simulink model "positionControlLoopCircle"  (Simulink 7.5)
settings: Solver=FixedStepDiscrete  StartTime=0.0  StopTime=Inf  FixedStep=Ts  RelTol=1e-3
PostLoadFcn:
  | , if any(exist('dsrtsu_mdlpostloadfcn', 'file') == [2, 3, 6]), try dsrtsu_mdlpostloadfcn('Execute', bdroot); catch fprintf('Error in PostLoadFcn (dsrtsu_mdlpostloadfcn) for model "%s":\n %s\n', bdroot, lasterr); end, end,
values from neighbouring files (symbols this model uses):
  Bx = 0.002015920056936    (= 0.00201592005694)    [main.m]
  By = 8.925446348616319e-004    (= 0.000892544634862)    [main.m]
  center = [xc;yc]    [main.m]    (also in main2.m)
  circX = center(1)+rad*cos(theta)    [genCircle.m]    (also in main.m = circXt(1:floor(length(circXt))); main2.m = circX(1:floor(length(circX)/factor)))
  circY = center(2)+rad*sin(theta)    [genCircle.m]    (also in main.m = circYt(1:floor(length(circYt))); main2.m = circY(1:floor(length(circY)/factor)))
  Jx = 9.170930148991473e-004    (= 0.000917093014899)    [main.m]
  Jy = 5.701918282653577e-004    (= 0.000570191828265)    [main.m]
  Ts = 0.01    [main.m]    (also in main2.m = 0.001)
  zeta = 0.8    [main.m]
undefined symbols (not defined in the file or in its folder): DiscIntNeverNeededParam
libraries: rtilib1103 x12, simulink x2
settings Model: DSRTSU_INTERNAL_RTI_VER=360  DSRTSU_INTERNAL_RTI_TYPE=rti1103  Creator=daq  LastModifiedBy=daq  BufferReuse=off
settings OptimizationCC: BlockReduction=off  OptimizeBlockIOStorage=off  BufferReuse=off  ExpressionFolding=off  LocalBlockOutputs=off
settings HardwareCC: ProdIntDivRoundTo=Zero  ProdEndianess=BigEndian  ProdHWDeviceType=Generic->Custom  TargetIntDivRoundTo=Zero  TargetEndianess=BigEndian  TargetHWDeviceType=Generic->Custom
settings RTWCC: SystemTargetFile=rti1103.tlc  MakeCommand=make_rti  TemplateMakefile=rti1103.tmf  Description=dSPACE DS1103 Hardware Platform  ProcessScript=rti1103_make_rtw_hook
settings STFCustomTargetCC: ParMdlRefBuildCompliant=on  GeneratePreprocessorConditionals=Disable all  SystemTargetFile=rti1103.tlc
settings GRTTargetCC: CompOptLevelCompliant=off  MatFileLogging=off  ExtModeMexFile=noextcomm
settings CustomProperty: DataType=RTWOptions_EnumType_C__dSPACE_matlab_rti1103_tlc_rti1103_1InitialSimState  Value=RUN
settings EnumStrPairs: String=RUN

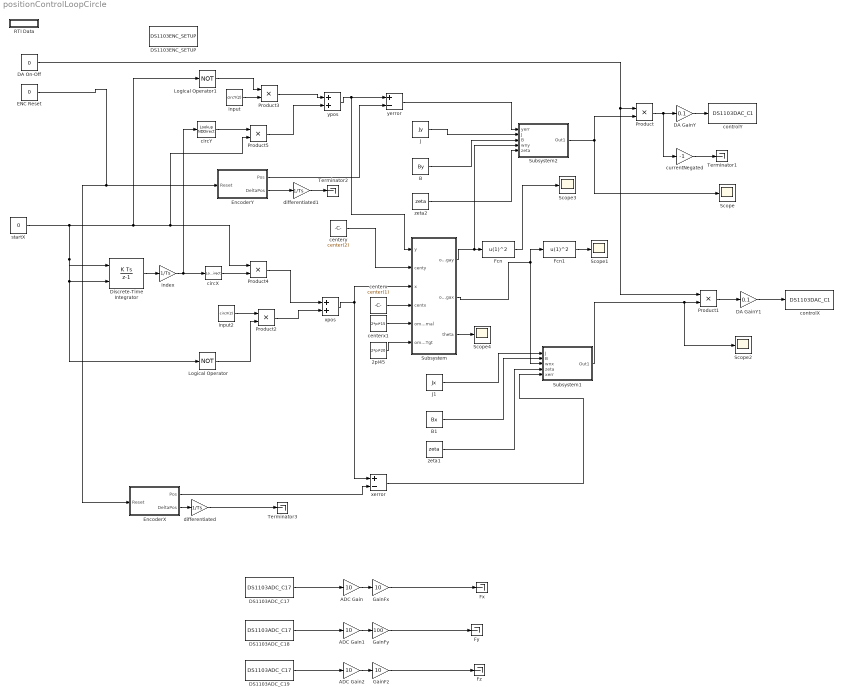
== system positionControlLoopCircle ==
  " EncoderX" : Subsystem
  " EncoderY" : Subsystem
  2pi45 : Constant  Value=2*pi*20  OutDataType=fixdt(1, 16)  OutScaling=2^0
  ADC Gain : Gain  Gain=10  ParameterDataType=fixdt(1, 16)  ParameterScaling=2^0  OutDataType=fixdt(1, 16)  OutScaling=2^0
  ADC Gain1 : Gain  Gain=10  ParameterDataType=fixdt(1, 16)  ParameterScaling=2^0  OutDataType=fixdt(1, 16)  OutScaling=2^0
  ADC Gain2 : Gain  Gain=10  ParameterDataType=fixdt(1, 16)  ParameterScaling=2^0  OutDataType=fixdt(1, 16)  OutScaling=2^0
  B : Constant  Value=By  OutDataType=fixdt(1, 16)  OutScaling=2^0
  B1 : Constant  Value=Bx  OutDataType=fixdt(1, 16)  OutScaling=2^0
  DA GainY : Gain  Gain=0.1  ParameterDataType=fixdt(1, 16)  ParameterScaling=2^0  OutDataType=fixdt(1, 16)  OutScaling=2^0
  DA GainY1 : Gain  Gain=0.1  ParameterDataType=fixdt(1, 16)  ParameterScaling=2^0  OutDataType=fixdt(1, 16)  OutScaling=2^0
  DA On-Off : Constant  Value=0  OutDataType=fixdt(1, 16)  OutScaling=2^0
  DS1103ADC_C17 : rtilib1103/DS1103 MASTER PPC/DS1103ADC_C17  SystemSampleTime=-1  ChannelNo=17  TimerAPreTrigger=0  Reserved2=[]  Reserved3=[]  Reserved4=[]  DialogFcn=gui1103adc  UnitName={ 'DS1103ADC_C' }  UnitValues={ 17 }  DSProperties=struct('RTI',struct('Version',uint32(1),'BlockType',struct('isSLSource',uint8(1),'isSLSink',uint8(0),'isHWSource',uint8(1),'isHWSink',uint8(0),'isSetup',uint8(0),'isInline',uint8(1),'isNonInline',uint8(0),'isInterrupt',uint8(0),'isChannelwise',uint8(1)),'IOBoardType','DS1103MASTER','UnitType','ADC','Identifier','ADC','DialogType','ML','BlockSet','NONE','SlaveProcessor','NONE'))
  DS1103ADC_C18 : rtilib1103/DS1103 MASTER PPC/DS1103ADC_C17  SystemSampleTime=-1  ChannelNo=18  TimerAPreTrigger=0  Reserved2=[]  Reserved3=[]  Reserved4=[]  DialogFcn=gui1103adc  UnitName={ 'DS1103ADC_C' }  UnitValues={ 18 }  DSProperties=struct('RTI',struct('Version',uint32(1),'BlockType',struct('isSLSource',uint8(1),'isSLSink',uint8(0),'isHWSource',uint8(1),'isHWSink',uint8(0),'isSetup',uint8(0),'isInline',uint8(1),'isNonInline',uint8(0),'isInterrupt',uint8(0),'isChannelwise',uint8(1)),'IOBoardType','DS1103MASTER','UnitType','ADC','Identifier','ADC','DialogType','ML','BlockSet','NONE','SlaveProcessor','NONE'))
  DS1103ADC_C19 : rtilib1103/DS1103 MASTER PPC/DS1103ADC_C17  SystemSampleTime=-1  ChannelNo=19  TimerAPreTrigger=0  Reserved2=[]  Reserved3=[]  Reserved4=[]  DialogFcn=gui1103adc  UnitName={ 'DS1103ADC_C' }  UnitValues={ 19 }  DSProperties=struct('RTI',struct('Version',uint32(1),'BlockType',struct('isSLSource',uint8(1),'isSLSink',uint8(0),'isHWSource',uint8(1),'isHWSink',uint8(0),'isSetup',uint8(0),'isInline',uint8(1),'isNonInline',uint8(0),'isInterrupt',uint8(0),'isChannelwise',uint8(1)),'IOBoardType','DS1103MASTER','UnitType','ADC','Identifier','ADC','DialogType','ML','BlockSet','NONE','SlaveProcessor','NONE'))
  DS1103ENC_SETUP : rtilib1103/DS1103 MASTER PPC/DS1103ENC_SETUP  SystemSampleTime=-1  EncRange=0  Reserved1=[]  Reserved2=[]  Reserved3=[]  Reserved4=[]  DialogFcn=gui1103enc_setup  UnitName={ 'DS1103ENC_SETUP' }  UnitValues={ [] }  DSProperties=struct('RTI',struct('Version',uint32(1),'BlockType',struct('isSLSource',uint8(0),'isSLSink',uint8(0),'isHWSource',uint8(0),'isHWSink',uint8(0),'isSetup',uint8(0),'isInline',uint8(1),'isNonInline',uint8(0),'isInterrupt',uint8(0),'isChannelwise',uint8(0)),'IOBoardType','DS1103MASTER','UnitType','ENC','Identifier','ENCMASTER','DialogType','ML','BlockSet','NONE','SlaveProcessor','NONE'))
      settings: SignalType=[0 0 0 0 0 0 0]
  Discrete-Time Integrator : DiscreteIntegrator  ExternalReset=rising  SampleTime=Ts  OutDataType=fixdt(1, 16)  OutScaling=2^0  ICPrevOutput=DiscIntNeverNeededParam  ICPrevScaledInput=DiscIntNeverNeededParam
  ENC Reset : Constant  Value=0  OutDataType=fixdt(1, 16)  OutScaling=2^0
  Fcn : Fcn  Expr=u(1)^2
  Fcn1 : Fcn  Expr=u(1)^2
  Fx : Terminator
  Fy : Terminator
  Fz : Terminator
  GainFx : Gain  Gain=10  ParameterDataType=fixdt(1, 16)  ParameterScaling=2^0  OutDataType=fixdt(1, 16)  OutScaling=2^0
  GainFy : Gain  Gain=100  ParameterDataType=fixdt(1, 16)  ParameterScaling=2^0  OutDataType=fixdt(1, 16)  OutScaling=2^0
  GainFz : Gain  Gain=10  ParameterDataType=fixdt(1, 16)  ParameterScaling=2^0  OutDataType=fixdt(1, 16)  OutScaling=2^0
  J : Constant  Value=Jy  OutDataType=fixdt(1, 16)  OutScaling=2^0
  J1 : Constant  Value=Jx  OutDataType=fixdt(1, 16)  OutScaling=2^0
  Logical Operator : Logic  Operator=NOT  AllPortsSameDT=off  OutDataTypeMode=boolean  LogicDataType=fixdt(0, 8)  OutDataTypeStr=boolean
  Logical Operator1 : Logic  Operator=NOT  AllPortsSameDT=off  OutDataTypeMode=boolean  LogicDataType=fixdt(0, 8)  OutDataTypeStr=boolean
  Product{,1..5} (6 alike) : Product  OutDataType=fixdt(1, 16)  OutScaling=2^0  RndMeth=Zero
  RTI Data : Subsystem  Tag=struct('RTIDataServer',struct('RTIDataServerVs','2','RTIModelDescription','struct(''main'',''positionControlLoopCircle'',''sub'','''',''isMp'',0)'))  LoadFcn="if exist('rtidc'), try,  rtidc('DataHostBlockClbLoad', gcbh); catch, disp(['Warning: ''LoadFcn'' for RTI Data block failed: ' lasterr]); end, end,"
      settings: CopyFcn="if exist('rtidc'), try,  rtidc('DataHostBlockClbCopy', gcbh); catch, disp(['Warning: ''CopyFcn'' for RTI Data block failed: ' lasterr]); end, end,"  DeleteFcn="if exist('rtidc'), try,  rtidc('DataHostBlockClbDelete', gcbh); catch, disp(['Warning: ''DeleteFcn'' for RTI Data block failed: ' lasterr]); end, end,"  ModelCloseFcn="if exist('rtidc'), try,  rtidc('DataHostBlockClbModelClose', gcbh); catch, disp(['Warning: ''ModelCloseFcn'' for RTI Data block failed: ' lasterr]); end, end,"  PreSaveFcn="if exist('rtidc'), try,  rtidc('DataHostBlockClbPreSave', gcbh); catch, disp(['Warning: ''PreSaveFcn'' for RTI Data block failed: ' lasterr]); end, end,"  PostSaveFcn="if exist('rtidc'), try,  rtidc('DataHostBlockClbPostSave', gcbh); catch, disp(['Warning: ''PostSaveFcn'' for RTI Data block failed: ' lasterr]); end, end,"  NameChangeFcn="if exist('rtidc'), try,  rtidc('DataHostBlockClbNameChange', gcbh); catch, disp(['Warning: ''NameChangeFcn'' for RTI Data block failed: ' lasterr]); end, end,"
      mask Type: RTI_DATA_HOST
      mask Description:
      | RTI Data Block.
      | This block is used by RTI to store internal model-dependent data.
      | Please keep this block on the root level of the model. Deleting this block will result in data loss.
      | 
      | NEVER DELETE OR COPY THIS BLOCK!
      mask Help:
      | RTI Data Block.
      | This block is used by RTI to store internal model-dependent data.
      | Please keep this block on the root level of the model. Deleting this block will result in data loss.
      | 
      | NEVER DELETE OR COPY THIS BLOCK!
      mask Display:
      | text(0.5, 0.5, 'RTI Data', 'HorizontalAlignment', 'center');
      | plot([1 0]);
  Scope{,1..4} (5 alike) : Scope
      Scope2 settings: SaveName=ScopeData2
      Scope3 settings: SaveName=ScopeData3
      Scope4 settings: SaveName=ScopeData4
  Subsystem : Subsystem
  Subsystem1 : Subsystem
  Subsystem2 : Subsystem
  Terminator1 : Terminator
  Terminator2 : Terminator
  Terminator3 : Terminator
  centerx : Constant  Value=center(1)  OutDataType=fixdt(1, 16)  OutScaling=2^0
  centerx1 : Constant  Value=2*pi*15  OutDataType=fixdt(1, 16)  OutScaling=2^0
  centery : Constant  Value=center(2)  OutDataType=fixdt(1, 16)  OutScaling=2^0
  circX : LookupNDDirect  NumberOfTableDimensions=1  Table=circX
  circY : LookupNDDirect  NumberOfTableDimensions=1  Table=circY
  controlX : rtilib1103/DS1103 MASTER PPC/DS1103DAC_C1  SystemSampleTime=-1  ChannelNo=1  InitValue=0  TermMode=0  TermValue=0  Reserved1=[]  Reserved2=[]  Reserved3=[]  Reserved4=[]  DialogFcn=gui1103dac  UnitName={ 'DS1103DAC_C' }  UnitValues={ 1 }  DSProperties=struct('RTI',struct('Version',uint32(1),'BlockType',struct('isSLSource',uint8(0),'isSLSink',uint8(1),'isHWSource',uint8(0),'isHWSink',uint8(1),'isSetup',uint8(0),'isInline',uint8(1),'isNonInline',uint8(0),'isInterrupt',uint8(0),'isChannelwise',uint8(1)),'IOBoardType','DS1103MASTER','UnitType','DAC','Identifier','DAC','DialogType','ML','BlockSet','NONE','SlaveProcessor','NONE'))
  controlY : rtilib1103/DS1103 MASTER PPC/DS1103DAC_C1  SystemSampleTime=-1  ChannelNo=2  InitValue=0  TermMode=1  TermValue=0  Reserved1=[]  Reserved2=[]  Reserved3=[]  Reserved4=[]  DialogFcn=gui1103dac  UnitName={ 'DS1103DAC_C' }  UnitValues={ 2 }  DSProperties=struct('RTI',struct('Version',uint32(1),'BlockType',struct('isSLSource',uint8(0),'isSLSink',uint8(1),'isHWSource',uint8(0),'isHWSink',uint8(1),'isSetup',uint8(0),'isInline',uint8(1),'isNonInline',uint8(0),'isInterrupt',uint8(0),'isChannelwise',uint8(1)),'IOBoardType','DS1103MASTER','UnitType','DAC','Identifier','DAC','DialogType','ML','BlockSet','NONE','SlaveProcessor','NONE'))
  currentNegated : Gain  Gain=-1  ParameterDataType=fixdt(1, 16)  ParameterScaling=2^0  OutDataType=fixdt(1, 16)  OutScaling=2^0
  differentiated : Gain  Gain=1/Ts  ParameterDataType=fixdt(1, 16)  ParameterScaling=2^0  OutDataType=fixdt(1, 16)  OutScaling=2^0
  differentiated1 : Gain  Gain=1/Ts  ParameterDataType=fixdt(1, 16)  ParameterScaling=2^0  OutDataType=fixdt(1, 16)  OutScaling=2^0
  index : Gain  Gain=1/Ts  ParameterDataType=fixdt(1, 16)  ParameterScaling=2^0  OutDataType=fixdt(1, 16)  OutScaling=2^0
  input : Constant  Value=circY(2)  OutDataType=fixdt(1, 16)  OutScaling=2^0
  input2 : Constant  Value=circX(2)  OutDataType=fixdt(1, 16)  OutScaling=2^0
  startX : Constant  Value=0  OutDataType=fixdt(1, 16)  OutScaling=2^0
  xerror : Sum  Inputs=+-  OutDataType=fixdt(1, 16)  OutScaling=2^-10
  xpos : Sum  OutDataType=fixdt(1, 16)  OutScaling=2^-10
  yerror : Sum  Inputs=+-  OutDataType=fixdt(1, 16)  OutScaling=2^-10
  ypos : Sum  OutDataType=fixdt(1, 16)  OutScaling=2^-10
  zeta1 : Constant  Value=zeta  OutDataType=fixdt(1, 16)  OutScaling=2^0
  zeta2 : Constant  Value=zeta  OutDataType=fixdt(1, 16)  OutScaling=2^0
  wires:
  " EncoderY"/1(Pos) -> yerror/2
  DA GainY/1 -> controlY/1
  Product/1 -> DA GainY/1, currentNegated/1
  DA On-Off/1 -> Product1/1, Product/1
  ENC Reset/1 -> " EncoderY"/1(Reset), " EncoderX"/1(Reset)
  DS1103ADC_C18/1 -> ADC Gain1/1
  GainFz/1 -> Fz/1
  DS1103ADC_C17/1 -> ADC Gain/1
  ADC Gain/1 -> GainFx/1
  ADC Gain1/1 -> GainFy/1
  ADC Gain2/1 -> GainFz/1
  GainFy/1 -> Fy/1
  currentNegated/1 -> Terminator1/1
  " EncoderX"/2(DeltaPos) -> differentiated/1
  " EncoderY"/2(DeltaPos) -> differentiated1/1
  GainFx/1 -> Fx/1
  DS1103ADC_C19/1 -> ADC Gain2/1
  startX/1 -> Discrete-Time Integrator/1, Discrete-Time Integrator/2, Logical Operator/1, Logical Operator1/1, Product4/1, Product5/2
  Discrete-Time Integrator/1 -> index/1
  index/1 -> circX/1, circY/1
  ypos/1 -> yerror/1, Subsystem/1(y)
  differentiated1/1 -> Terminator2/1
  differentiated/1 -> Terminator3/1
  Subsystem2/1(Out1) -> Product/2, Scope/1
  centery/1 -> Subsystem/2(centy)
  centerx/1 -> Subsystem/4(centx)
  2pi45/1 -> Subsystem/6(omegaTgt)
  xpos/1 -> Subsystem/3(x), xerror/1
  " EncoderX"/1(Pos) -> xerror/2
  Subsystem1/1(Out1) -> Product1/2, Scope2/1
  Product1/1 -> DA GainY1/1
  DA GainY1/1 -> controlX/1
  Subsystem/1(omegay) -> Subsystem2/4(wny), Fcn/1
  Subsystem/2(omegax) -> Subsystem1/3(wnx), Fcn1/1
  centerx1/1 -> Subsystem/5(omegaNormal)
  Subsystem/3(theta) -> Scope4/1
  J1/1 -> Subsystem1/1(J)
  B1/1 -> Subsystem1/2(B)
  xerror/1 -> Subsystem1/5(xerr)
  zeta1/1 -> Subsystem1/4(zeta)
  J/1 -> Subsystem2/2(J)
  B/1 -> Subsystem2/3(B)
  zeta2/1 -> Subsystem2/5(zeta)
  yerror/1 -> Subsystem2/1(yerr)
  Fcn/1 -> Scope3/1
  Fcn1/1 -> Scope1/1
  input2/1 -> Product2/1
  Product2/1 -> xpos/2
  Logical Operator/1 -> Product2/2
  input/1 -> Product3/2
  Product3/1 -> ypos/1
  Logical Operator1/1 -> Product3/1
  circX/1 -> Product4/2
  Product4/1 -> xpos/1
  circY/1 -> Product5/1
  Product5/1 -> ypos/2

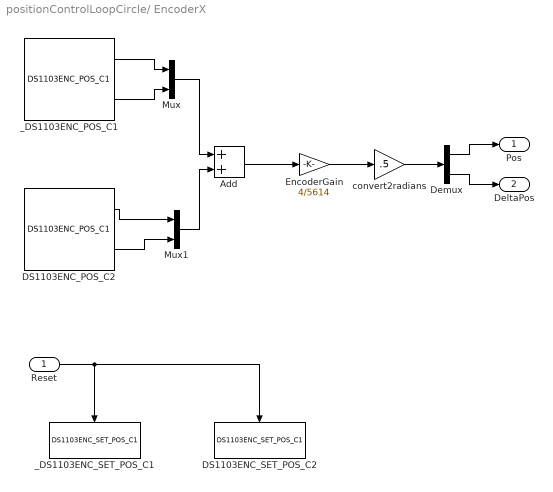
== system positionControlLoopCircle/ EncoderX ==
  Reset : Inport
  Add : Sum  OutDataType=fixdt(1, 16)  OutScaling=2^-10
  DS1103ENC_POS_C2 : rtilib1103/DS1103 MASTER PPC/DS1103ENC_POS_C1  SystemSampleTime=-1  ChannelNo=2  PosValue=0  Reserved1=[]  Reserved2=[]  Reserved3=[]  Reserved4=[]  DialogFcn=gui1103enc_pos  UnitName={ 'DS1103ENC_POS_C' }  UnitValues={ 2 }  DSProperties=struct('RTI',struct('Version',uint32(1),'BlockType',struct('isSLSource',uint8(1),'isSLSink',uint8(0),'isHWSource',uint8(1),'isHWSink',uint8(0),'isSetup',uint8(0),'isInline',uint8(1),'isNonInline',uint8(0),'isInterrupt',uint8(0),'isChannelwise',uint8(1)),'IOBoardType','DS1103MASTER','UnitType','ENC','Identifier','ENCPOSCH','DialogType','ML','BlockSet','NONE','SlaveProcessor','NONE'))
  DS1103ENC_SET_POS_C2 : rtilib1103/DS1103 MASTER PPC/DS1103ENC_SET_POS_C1  SystemSampleTime=-1  ChannelNo=2  PosValue=0  Reserved1=[]  Reserved2=[]  Reserved3=[]  Reserved4=[]  DialogFcn=gui1103enc_set_pos  UnitName={ 'DS1103ENC_SET_POS_C' }  UnitValues={ 2 }  DSProperties=struct('RTI',struct('Version',uint32(1),'BlockType',struct('isSLSource',uint8(0),'isSLSink',uint8(1),'isHWSource',uint8(0),'isHWSink',uint8(1),'isSetup',uint8(0),'isInline',uint8(1),'isNonInline',uint8(0),'isInterrupt',uint8(0),'isChannelwise',uint8(1)),'IOBoardType','DS1103MASTER','UnitType','ENC','Identifier','ENCRESET','DialogType','ML','BlockSet','NONE','SlaveProcessor','NONE'))
  Demux : Demux  Outputs=2
  EncoderGain : Gain  Gain=4/5614  SaturateOnIntegerOverflow=on  OutDataTypeStr=Inherit: Same as input  ParamDataTypeStr=Inherit: Same as input
  Mux : Mux  Inputs=2
  Mux1 : Mux  Inputs=2
  _DS1103ENC_POS_C1 : rtilib1103/DS1103 MASTER PPC/DS1103ENC_POS_C1  SystemSampleTime=-1  ChannelNo=1  PosValue=0  Reserved1=[]  Reserved2=[]  Reserved3=[]  Reserved4=[]  DialogFcn=gui1103enc_pos  UnitName={ 'DS1103ENC_POS_C' }  UnitValues={ 1 }  DSProperties=struct('RTI',struct('Version',uint32(1),'BlockType',struct('isSLSource',uint8(1),'isSLSink',uint8(0),'isHWSource',uint8(1),'isHWSink',uint8(0),'isSetup',uint8(0),'isInline',uint8(1),'isNonInline',uint8(0),'isInterrupt',uint8(0),'isChannelwise',uint8(1)),'IOBoardType','DS1103MASTER','UnitType','ENC','Identifier','ENCPOSCH','DialogType','ML','BlockSet','NONE','SlaveProcessor','NONE'))
  _DS1103ENC_SET_POS_C1 : rtilib1103/DS1103 MASTER PPC/DS1103ENC_SET_POS_C1  SystemSampleTime=-1  ChannelNo=1  PosValue=0  Reserved1=[]  Reserved2=[]  Reserved3=[]  Reserved4=[]  DialogFcn=gui1103enc_set_pos  UnitName={ 'DS1103ENC_SET_POS_C' }  UnitValues={ 1 }  DSProperties=struct('RTI',struct('Version',uint32(1),'BlockType',struct('isSLSource',uint8(0),'isSLSink',uint8(1),'isHWSource',uint8(0),'isHWSink',uint8(1),'isSetup',uint8(0),'isInline',uint8(1),'isNonInline',uint8(0),'isInterrupt',uint8(0),'isChannelwise',uint8(1)),'IOBoardType','DS1103MASTER','UnitType','ENC','Identifier','ENCRESET','DialogType','ML','BlockSet','NONE','SlaveProcessor','NONE'))
  "convert2radians " : Gain  Gain=.5
  Pos : Outport
  DeltaPos : Outport  Port=2
  wires:
  _DS1103ENC_POS_C1/1 -> Mux/1
  _DS1103ENC_POS_C1/2 -> Mux/2
  EncoderGain/1 -> "convert2radians "/1
  "convert2radians "/1 -> Demux/1
  Reset/1 -> _DS1103ENC_SET_POS_C1/Trigger, DS1103ENC_SET_POS_C2/Trigger
  Mux/1 -> Add/1
  Demux/1 -> Pos/1
  Demux/2 -> DeltaPos/1
  Mux1/1 -> Add/2
  DS1103ENC_POS_C2/1 -> Mux1/1
  DS1103ENC_POS_C2/2 -> Mux1/2
  Add/1 -> EncoderGain/1

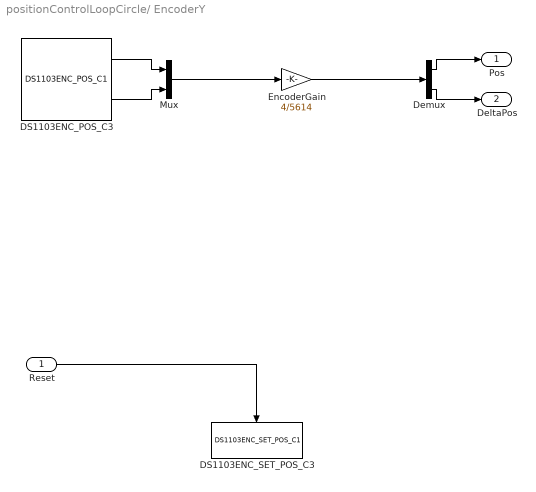
== system positionControlLoopCircle/ EncoderY ==
  Reset : Inport
  DS1103ENC_POS_C3 : rtilib1103/DS1103 MASTER PPC/DS1103ENC_POS_C1  SystemSampleTime=-1  ChannelNo=3  PosValue=0  Reserved1=[]  Reserved2=[]  Reserved3=[]  Reserved4=[]  DialogFcn=gui1103enc_pos  UnitName={ 'DS1103ENC_POS_C' }  UnitValues={ 3 }  DSProperties=struct('RTI',struct('Version',uint32(1),'BlockType',struct('isSLSource',uint8(1),'isSLSink',uint8(0),'isHWSource',uint8(1),'isHWSink',uint8(0),'isSetup',uint8(0),'isInline',uint8(1),'isNonInline',uint8(0),'isInterrupt',uint8(0),'isChannelwise',uint8(1)),'IOBoardType','DS1103MASTER','UnitType','ENC','Identifier','ENCPOSCH','DialogType','ML','BlockSet','NONE','SlaveProcessor','NONE'))
  DS1103ENC_SET_POS_C3 : rtilib1103/DS1103 MASTER PPC/DS1103ENC_SET_POS_C1  SystemSampleTime=-1  ChannelNo=3  PosValue=0  Reserved1=[]  Reserved2=[]  Reserved3=[]  Reserved4=[]  DialogFcn=gui1103enc_set_pos  UnitName={ 'DS1103ENC_SET_POS_C' }  UnitValues={ 3 }  DSProperties=struct('RTI',struct('Version',uint32(1),'BlockType',struct('isSLSource',uint8(0),'isSLSink',uint8(1),'isHWSource',uint8(0),'isHWSink',uint8(1),'isSetup',uint8(0),'isInline',uint8(1),'isNonInline',uint8(0),'isInterrupt',uint8(0),'isChannelwise',uint8(1)),'IOBoardType','DS1103MASTER','UnitType','ENC','Identifier','ENCRESET','DialogType','ML','BlockSet','NONE','SlaveProcessor','NONE'))
  Demux : Demux  Outputs=2
  EncoderGain : Gain  Gain=4/5614  SaturateOnIntegerOverflow=on  OutDataTypeStr=Inherit: Same as input  ParamDataTypeStr=Inherit: Same as input
  Mux : Mux  Inputs=2
  Pos : Outport
  DeltaPos : Outport  Port=2
  wires:
  Mux/1 -> EncoderGain/1
  Demux/2 -> DeltaPos/1
  Demux/1 -> Pos/1
  Reset/1 -> DS1103ENC_SET_POS_C3/Trigger
  EncoderGain/1 -> Demux/1
  DS1103ENC_POS_C3/2 -> Mux/2
  DS1103ENC_POS_C3/1 -> Mux/1

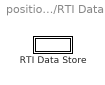
== system positionControlLoopCircle/RTI Data ==
  RTI Data Store : Subsystem  Tag="struct('private',struct('version',struct('dsVer',uint32(2),'dsVerCreation',uint32(2),'RTI',struct('ver','6.5','type','RTI1103')),'access',struct('type','Model','isPerm',1,'created',['16-Oct-2016 18:11:40'],'modified',['23-Jan-2017 23:02:30'],'location','')),'public',struct('main',struct('data',[]),'sub',struct('name',{{'positionControlLoopCircle'}},'data',{{struct('TH',struct('thTaskInfo',struct('taskType',{'TIMER','HWINT','TMRINT','SWINT'},'tasksNumOf',{1,0,0,0},'srcIds',{{'TIMERA'},{},{},{}},'taskNames',{{['Timer Task 1']},{},{},{}})),'th_tc',struct('dataType','TASK','taskGroupId','','taskGroupList',{{}},'taskSchedulingPolicy','FCFS','taskType','TIMER','blkh',-1,'srcId','TIMERA','srcSgnName',['Timer A interrupt'],'srcCpuName','','taskName',['Timer Task 1  [0.01] s'],'taskNameDisplayExt','','smplTime',0.01,'smplTimeOffs',0,'hasFixedPriority',0,'priority',1,'hasFixedOvc',0,'ovcType',1,'ovcMax',1),'tc_th',struct('dataType','TASK','taskGroupId','','taskGroupList',{{}},'taskSchedulingPolicy','FCFS','taskType','TIMER','blkh',-1,'srcId','TIMERA','srcSgnName',['Timer A interrupt'],'srcCpuName','','taskName',['Timer Task 1  [0.01] s'],'taskNameDisplayExt','','smplTime',0.01,'smplTimeOffs',0,'hasFixedPriority',0,'priority',1,'hasFixedOvc',0,'ovcType',1,'ovcMax',1))}})))"
      mask Type: RTI_DATA_STORE
      mask Description:
      | RTI Data Store Block. This block is used by RTI to store internal model dependent data. Deleting this block will result in data loss.
      | 
      | NEVER DELETE, COPY, OR MODIFY THIS BLOCK!
      mask Help:
      | RTI Data Store Block. This block is used by RTI to store internal model dependent data. Deleting this block will result in data loss.
      | 
      | NEVER DELETE, COPY, OR MODIFY THIS BLOCK!
      mask Display: text(0.5, 0.5, ' ', 'HorizontalAlignment', 'center');

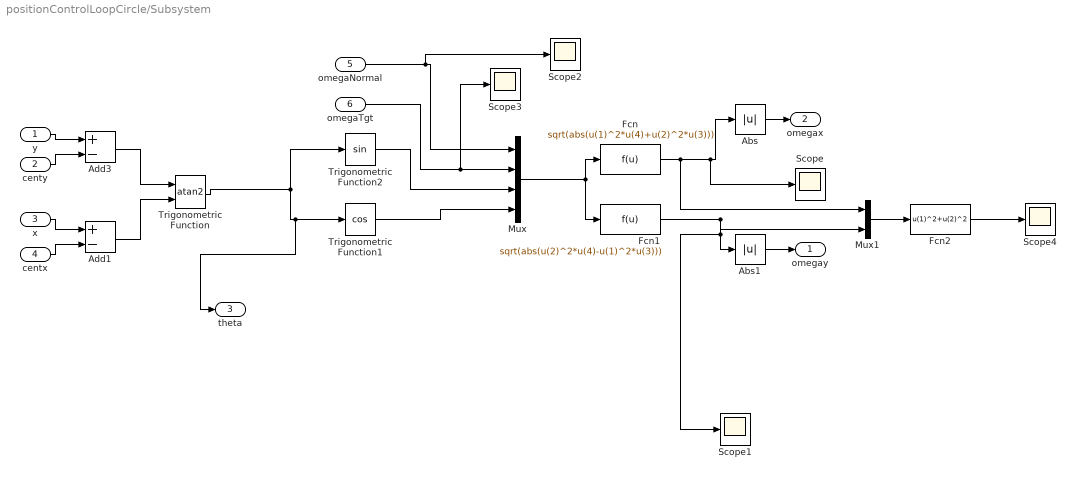
== system positionControlLoopCircle/Subsystem ==
  y : Inport
  centy : Inport  Port=2
  x : Inport  Port=3
  centx : Inport  Port=4
  omegaNormal : Inport  Port=5  OutDataType=fixdt(1, 16)  OutScaling=2^0
  omegaTgt : Inport  Port=6  OutDataType=fixdt(1, 16)  OutScaling=2^0
  Abs : Abs  OutDataType=fixdt(1, 16)  OutScaling=2^0
  Abs1 : Abs  OutDataType=fixdt(1, 16)  OutScaling=2^0
  Add1 : Sum  Inputs=+-  OutDataType=fixdt(1, 16)  OutScaling=2^-10
  Add3 : Sum  Inputs=+-  OutDataType=fixdt(1, 16)  OutScaling=2^-10
  Fcn : Fcn  Expr=sqrt(abs(u(1)^2*u(4)+u(2)^2*u(3)))
  Fcn1 : Fcn  Expr=sqrt(abs(u(2)^2*u(4)-u(1)^2*u(3)))
  Fcn2 : Fcn  Expr=u(1)^2+u(2)^2
  Mux : Mux
  Mux1 : Mux  Inputs=2
  Scope{,1..4} (5 alike) : Scope
      Scope settings: SaveName=ScopeData5
      Scope1 settings: SaveName=ScopeData6
      Scope2 settings: SaveName=ScopeData7
      Scope3 settings: SaveName=ScopeData8
      Scope4 settings: SaveName=ScopeData9
  Trigonometric Function : Trigonometry  Operator=atan2
  Trigonometric Function1 : Trigonometry  Operator=cos
  Trigonometric Function2 : Trigonometry
  omegay : Outport  OutDataType=fixdt(1, 16)  OutScaling=2^0
  omegax : Outport  Port=2  OutDataType=fixdt(1, 16)  OutScaling=2^0
  theta : Outport  Port=3  OutDataType=fixdt(1, 16)  OutScaling=2^0
  wires:
  x/1 -> Add1/1
  centx/1 -> Add1/2
  y/1 -> Add3/1
  centy/1 -> Add3/2
  Trigonometric Function/1 -> Trigonometric Function2/1, Trigonometric Function1/1, theta/1
  Add3/1 -> Trigonometric Function/1
  Add1/1 -> Trigonometric Function/2
  omegaNormal/1 -> Mux/1, Scope2/1
  omegaTgt/1 -> Mux/2, Scope3/1
  Trigonometric Function2/1 -> Mux/3
  Trigonometric Function1/1 -> Mux/4
  Mux/1 -> Fcn/1, Fcn1/1
  Fcn/1 -> Abs/1, Scope/1, Mux1/1
  Fcn1/1 -> Abs1/1, Scope1/1, Mux1/2
  Abs/1 -> omegax/1
  Abs1/1 -> omegay/1
  Mux1/1 -> Fcn2/1
  Fcn2/1 -> Scope4/1

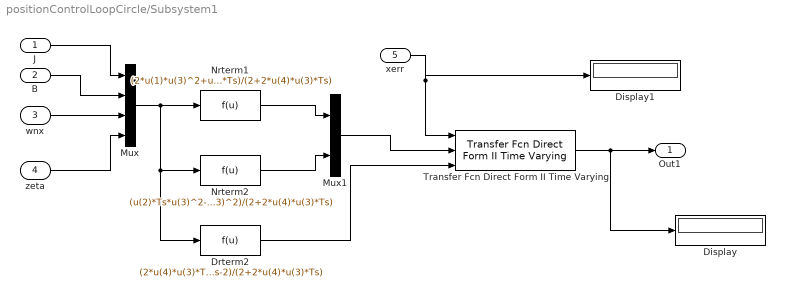
== system positionControlLoopCircle/Subsystem1 ==
  J : Inport
  B : Inport  Port=2
  wnx : Inport  Port=3
  zeta : Inport  Port=4
  xerr : Inport  Port=5
  Display : Display
  Display1 : Display
  Drterm2 : Fcn  Expr=(2*u(4)*u(3)*Ts-2)/(2+2*u(4)*u(3)*Ts)
  Mux : Mux
  Mux1 : Mux  Inputs=2
  Nrterm1 : Fcn  Expr=(2*u(1)*u(3)^2+u(2)*u(3)^2*Ts)/(2+2*u(4)*u(3)*Ts)
  Nrterm2 : Fcn  Expr=(u(2)*Ts*u(3)^2-2*u(1)*u(3)^2)/(2+2*u(4)*u(3)*Ts)
  Transfer Fcn Direct Form II Time Varying : simulink/Additional Math & Discrete/Additional Discrete/Transfer Fcn Direct Form II Time Varying  SystemSampleTime=-1  vinit=0.0  DoSatur=off
  Out1 : Outport  OutDataType=fixdt(1, 16)  OutScaling=2^0
  wires:
  J/1 -> Mux/1
  wnx/1 -> Mux/3
  Mux/1 -> Nrterm1/1, Nrterm2/1, Drterm2/1
  zeta/1 -> Mux/4
  B/1 -> Mux/2
  Nrterm1/1 -> Mux1/1
  Nrterm2/1 -> Mux1/2
  Mux1/1 -> Transfer Fcn Direct Form II Time Varying/2
  xerr/1 -> Transfer Fcn Direct Form II Time Varying/1, Display1/1
  Drterm2/1 -> Transfer Fcn Direct Form II Time Varying/3
  Transfer Fcn Direct Form II Time Varying/1 -> Out1/1, Display/1

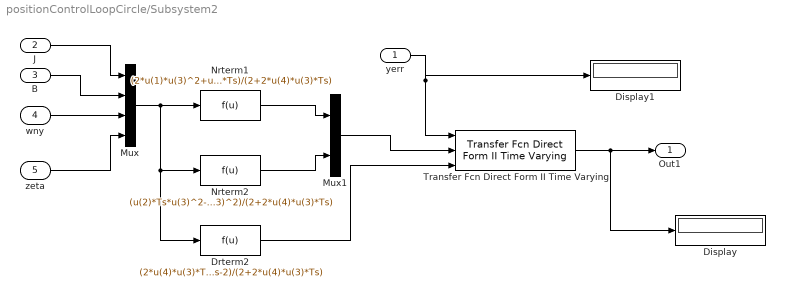
== system positionControlLoopCircle/Subsystem2 ==
  yerr : Inport
  J : Inport  Port=2
  B : Inport  Port=3
  wny : Inport  Port=4
  zeta : Inport  Port=5
  Display : Display
  Display1 : Display
  Drterm2 : Fcn  Expr=(2*u(4)*u(3)*Ts-2)/(2+2*u(4)*u(3)*Ts)
  Mux : Mux
  Mux1 : Mux  Inputs=2
  Nrterm1 : Fcn  Expr=(2*u(1)*u(3)^2+u(2)*u(3)^2*Ts)/(2+2*u(4)*u(3)*Ts)
  Nrterm2 : Fcn  Expr=(u(2)*Ts*u(3)^2-2*u(1)*u(3)^2)/(2+2*u(4)*u(3)*Ts)
  Transfer Fcn Direct Form II Time Varying : simulink/Additional Math & Discrete/Additional Discrete/Transfer Fcn Direct Form II Time Varying  SystemSampleTime=-1  vinit=0.0  DoSatur=off
  Out1 : Outport  OutDataType=fixdt(1, 16)  OutScaling=2^0
  wires:
  Transfer Fcn Direct Form II Time Varying/1 -> Display/1, Out1/1
  Drterm2/1 -> Transfer Fcn Direct Form II Time Varying/3
  yerr/1 -> Display1/1, Transfer Fcn Direct Form II Time Varying/1
  Mux1/1 -> Transfer Fcn Direct Form II Time Varying/2
  Nrterm2/1 -> Mux1/2
  Nrterm1/1 -> Mux1/1
  B/1 -> Mux/2
  zeta/1 -> Mux/4
  Mux/1 -> Drterm2/1, Nrterm2/1, Nrterm1/1
  wny/1 -> Mux/3
  J/1 -> Mux/1

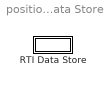
== system positionControlLoopCircle/RTI Data/RTI Data Store ==
  RTI Data Store : Subsystem
      mask Type: RTI_DATA_STORE
      mask Description:
      | RTI Data Store Block. This block is used by RTI to store internal model dependent data. Deleting this block will result in data loss.
      | 
      | NEVER DELETE, COPY, OR MODIFY THIS BLOCK!
      mask Help:
      | RTI Data Store Block. This block is used by RTI to store internal model dependent data. Deleting this block will result in data loss.
      | 
      | NEVER DELETE, COPY, OR MODIFY THIS BLOCK!
      mask Display: text(0.5, 0.5, ' ', 'HorizontalAlignment', 'center');

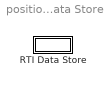
== system positionControlLoopCircle/RTI Data/RTI Data Store/RTI Data Store ==
  RTI Data Store : Subsystem
      mask Type: RTI_DATA_STORE
      mask Description:
      | RTI Data Store Block. This block is used by RTI to store internal model dependent data. Deleting this block will result in data loss.
      | 
      | NEVER DELETE, COPY, OR MODIFY THIS BLOCK!
      mask Help:
      | RTI Data Store Block. This block is used by RTI to store internal model dependent data. Deleting this block will result in data loss.
      | 
      | NEVER DELETE, COPY, OR MODIFY THIS BLOCK!
      mask Display: text(0.5, 0.5, ' ', 'HorizontalAlignment', 'center');

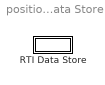
== system positionControlLoopCircle/RTI Data/RTI Data Store/RTI Data Store/RTI Data Store ==
  RTI Data Store : Subsystem
      mask Type: RTI_DATA_STORE
      mask Description:
      | RTI Data Store Block. This block is used by RTI to store internal model dependent data. Deleting this block will result in data loss.
      | 
      | NEVER DELETE, COPY, OR MODIFY THIS BLOCK!
      mask Help:
      | RTI Data Store Block. This block is used by RTI to store internal model dependent data. Deleting this block will result in data loss.
      | 
      | NEVER DELETE, COPY, OR MODIFY THIS BLOCK!
      mask Display: text(0.5, 0.5, ' ', 'HorizontalAlignment', 'center');

== system positionControlLoopCircle/RTI Data/RTI Data Store/RTI Data Store/RTI Data Store/RTI Data Store ==
